simulink library "PaperLib"  (R2024b)
settings: Solver=VariableStepAuto  StartTime=0.0  StopTime=10.0  RelTol=1e-3
libraries: NSA_DEVS_LOGISTICS x2, NSA_DEVS_MATH_OPERATIONS x1, NSA_DEVS_SINKS x1
settings Model: Creator=peter  LastModifiedBy=peter
settings RTWCC: GPUComputeCapability=3.5

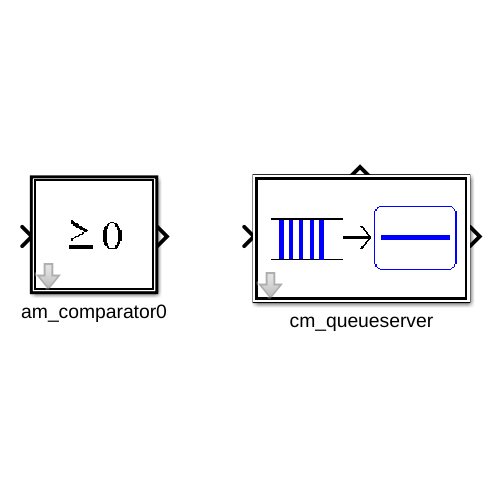
[thumbnail: Simulink's stored preview of the top-level diagram]
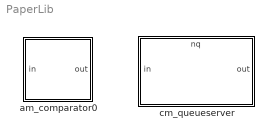
== system PaperLib ==
  am_comparator0 : Subsystem  TreatAsAtomicUnit=on  mask(Comparator){tau=[0,1], debug=0}
      mask help: Returns 1 if in >= 0, else 0.
      mask Help:
      | <p>Returns 1 if in >= 0, else 0.</p>
      | 
      | <p>Ports
      | <ul>
      | <li>inputs:
      |   <ul>
      |     <li>in: incoming value</li>
      |   </ul>
      | </li>
      | <li>outputs:
      |   <ul>
      |     <li>out: result value</li>
      |   </ul>
      | </li>
      | </ul>
      | </p>
      | 
      | <p>System Parameters
      | <ul>
      | <li>debug: flag to enable debug information</li>
      | <li>tau:   infinitesimal delay</li>
      | </ul>
      | </p>
      | 
      | <p>States
      | <ul>
      | <li>s:   running</li>
      | </ul>
      | </p>
      mask DialogControl Container6 Prompt: Advanced
      mask Display: image('$imagefile'); % Use "Edit Image" on toolstrip to change.
  cm_queueserver : Subsystem  mask{ts=4.5, tau=[0,1], debug=0}
      settings: PortSchema="{\"entries\":[{\"content\":{\"sides\":[{\"content\":{\"connectorIds\":[\"In1\"]},\"type\":\"ConnectorPlacement.EquallySpacedRectSide\",\"uuid\":\"07fa0e51-8843-4ac9-8e94-884ae9a89d36\"},{\"content\":{\"connectorIds\":[\"Out1\"],\"side\":\"RIGHT\"},\"type\":\"ConnectorPlacement.EquallySpacedRectSide\",\"uuid\":\"0131ce69-7449-4362-9cfd-88c0df269334\"},{\"content\":{\"connectorIds\":[\"Out2\"],\"side\":\"TOP\"},\"type\":\"ConnectorPlacement.EquallySpacedRectSide\",\"uuid\":\"407e2fdf-9916-4f3f-84c2-2a472bd1d59f\"}]},\"type\":\"ConnectorPlacement.EquallySpacedConnector\",\"uuid\":\"291a1c46-4425-425c-bba8-593c7bd17cc2\"}],\"packageUris\":[\"http://schema.mathworks.com/mf0/Connector/R2020b\"],\"version\":\"1.0\"}"
      mask DialogControl Container4 Prompt: General
      mask DialogControl Container5 Prompt: Advanced
      mask Display: image('$imagefile'); % Use "Edit Image" on toolstrip to change.

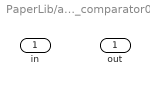
== system PaperLib/am_comparator0 ==
  in : Inport
  out : Outport

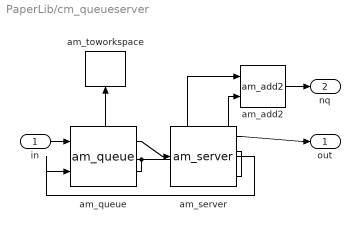
== system PaperLib/cm_queueserver ==
  in : Inport
  am_add2 : NSA_DEVS_MATH_OPERATIONS/am_add2  tau=tau  debug=debug
      settings: SourceProductName=Math Operations
  am_queue : NSA_DEVS_LOGISTICS/am_queue  tD=tau.*2  tau=tau  debug=debug
      settings: SourceProductName=Logistics
  am_server : NSA_DEVS_LOGISTICS/am_server  tS=ts  tsField="\"\""  tau=tau  debug=debug
      settings: SourceProductName=Logistics
  am_toworkspace : NSA_DEVS_SINKS/am_toworkspace  varname="\"nq1\""  t0=0  format="\"vector\""  tau=[0,5]  debug=0
      settings: SourceProductName=Sinks
  out : Outport
  nq : Outport  Port=2
  wires:
  am_add2/1 -> nq/1
  am_server/3 -> am_add2/2
  am_queue/2 -> am_toworkspace/1, am_add2/1
  am_server/1 -> out/1
  am_server/2 -> am_queue/2
  in/1 -> am_queue/1
  am_queue/1 -> am_server/1
